simulink model "simRobotArmWith2Links"  (R2014b)
settings: Solver=ode5  StartTime=0.0  StopTime=tf  FixedStep=dt  MaxStep=dtmax  RelTol=1e-3
values from neighbouring files (symbols this model uses):
  alpha = 1    [robotArmWith2Links.m]    (also in threeLinkFTC.m; twoLinkFTC.m; twoLinkFTCwAdaptive.m)
  Ar = [0 5; -30 -30]    [robotArmWith2Links.m]    (also in threeLinkFTC.m = [0 1; -5 -5]; twoLinkFTC.m = [0 10; -40 -40]; twoLinkFTCwAdaptive.m = [0 5; -250 -250])
  Arm1 = [0 1; -wn^2 -2*ksi*wn]    [robotArmWith2Links.m]    (also in threeLinkFTC.m; twoLinkFTC.m; twoLinkFTCwAdaptive.m)
  Bfault = [0 0; 0 1]    [robotArmWith2Links.m]    (also in threeLinkFTC.m; twoLinkFTC.m; twoLinkFTCwAdaptive.m)
  Brm1 = [0 wn^2]'    [robotArmWith2Links.m]    (also in threeLinkFTC.m; twoLinkFTC.m; twoLinkFTCwAdaptive.m)
  dt = 1e-3    (= 0.001)    [robotArmWith2Links.m]
  dtFC = dt    (= 0.001)    [robotArmWith2Links.m]
  epsilon = 0.5    [robotArmWith2Links.m]    (also in threeLinkFTC.m; twoLinkFTC.m; twoLinkFTCwAdaptive.m)
  g = 9.81    [robotArmWith2Links.m]    (also in threeLinkFTC.m; twoLinkFDIbasisComparison.m; twoLinkFTC.m; twoLinkFTCwAdaptive.m)
  I1 = 8.33e-2    (= 0.0833)    [robotArmWith2Links.m]    (also in threeLinkFTC.m = 0.0833333333333; twoLinkFDIbasisComparison.m = 0.0833333333333; twoLinkFTC.m = 0.0833333333333; twoLinkFTCwAdaptive.m = 0.0833333333333)
  I2 = 8.33e-2    (= 0.0833)    [robotArmWith2Links.m]    (also in threeLinkFTC.m = 0.0833333333333; twoLinkFDIbasisComparison.m = 0.0833333333333; twoLinkFTC.m = 0.0833333333333; twoLinkFTCwAdaptive.m = 0.0833333333333)
  K1 = 2*wn*ksi    (= 87.9645943005)    [robotArmWith2Links.m]    (also in threeLinkFTC.m = 8.79645943005; twoLinkFTC.m; twoLinkFTCwAdaptive.m = 43.9822971503)
  K2 = wn^2    (= 986.960440109)    [robotArmWith2Links.m]    (also in threeLinkFTC.m = 39.4784176044; twoLinkFTC.m; twoLinkFTCwAdaptive.m)
  l1 = 1    [robotArmWith2Links.m]    (also in threeLinkFTC.m; twoLinkFDIbasisComparison.m; twoLinkFTC.m; twoLinkFTCwAdaptive.m)
  l2 = 1    [robotArmWith2Links.m]    (also in threeLinkFTC.m; twoLinkFDIbasisComparison.m; twoLinkFTC.m; twoLinkFTCwAdaptive.m)
  lc1 = l1/2    (= 0.5)    [robotArmWith2Links.m]    (also in threeLinkFTC.m; twoLinkFDIbasisComparison.m; twoLinkFTC.m; twoLinkFTCwAdaptive.m)
  lc2 = l2/2    (= 0.5)    [robotArmWith2Links.m]    (also in threeLinkFTC.m; twoLinkFDIbasisComparison.m; twoLinkFTC.m; twoLinkFTCwAdaptive.m)
  m1 = 1    [robotArmWith2Links.m]    (also in threeLinkFTC.m; twoLinkFDIbasisComparison.m; twoLinkFTC.m; twoLinkFTCwAdaptive.m)
  m2 = 1    [robotArmWith2Links.m]    (also in threeLinkFTC.m; twoLinkFDIbasisComparison.m; twoLinkFTC.m; twoLinkFTCwAdaptive.m)
  q0 = [80 20]'*pi/180    [robotArmWith2Links.m]    (also in threeLinkFTC.m = [90 0 0]'*pi/180; twoLinkFDIbasisComparison.m = [90 0]'*pi/180; twoLinkFTC.m = [90 0]'*pi/180; twoLinkFTCwAdaptive.m = [90 0]'*pi/180)
  qdot0 = [0 0]'    [robotArmWith2Links.m]    (also in threeLinkFTC.m = [0 0 0]'*pi/180; twoLinkFDIbasisComparison.m = [0 0]'*pi/180; twoLinkFTC.m = [0 0]'*pi/180; twoLinkFTCwAdaptive.m = [0 0]'*pi/180)
  r0 = [0 0]'    [robotArmWith2Links.m]    (also in threeLinkFTC.m; twoLinkFTC.m; twoLinkFTCwAdaptive.m)
  rmax = inf*[50*pi/180 inf]'    [robotArmWith2Links.m]    (also in threeLinkFTC.m; twoLinkFTC.m; twoLinkFTCwAdaptive.m)
  rmin = -rmax    [robotArmWith2Links.m]    (also in threeLinkFTC.m; twoLinkFTC.m; twoLinkFTCwAdaptive.m)
  visualFlag = 0    [robotArmWith2Links.m]    (also in twoLinkFDIbasisComparison.m; twoLinkFTC.m; twoLinkFTCwAdaptive.m)
  visualizationDataFlag = 1    [robotArmWith2Links.m]    (also in twoLinkFDIbasisComparison.m; twoLinkFTC.m; twoLinkFTCwAdaptive.m)
undefined symbols (not defined in the file or in its folder): twolinkplot
libraries: simulink x1
(part 2 of 2)

== system simRobotArmWith2Links/Controller/ FTC Controller/System model/Modelled Plant/get Plant Parameters ==
  H : Inport
  C : Inport  Port=2
  G : Inport  Port=3
  qdot : Inport  Port=4
  {1,5,7,11} (4 alike) : Selector  NumberOfDimensions=2  InputPortWidth=3  IndexOptions=Index vector (dialog),Index vector (dialog)  Indices=1,1  OutputSizes=1,1
  12 : Selector  NumberOfDimensions=2  InputPortWidth=3  IndexOptions=Index vector (dialog),Index vector (dialog)  Indices=1,2  OutputSizes=1,1
  2 : Selector  NumberOfDimensions=2  InputPortWidth=3  IndexOptions=Index vector (dialog),Index vector (dialog)  Indices=1,2  OutputSizes=1,1
  {3,6,8,21} (4 alike) : Selector  NumberOfDimensions=2  InputPortWidth=3  IndexOptions=Index vector (dialog),Index vector (dialog)  Indices=2,1  OutputSizes=1,1
  22 : Selector  NumberOfDimensions=2  InputPortWidth=3  IndexOptions=Index vector (dialog),Index vector (dialog)  Indices=2,2  OutputSizes=1,1
  4 : Selector  NumberOfDimensions=2  InputPortWidth=3  IndexOptions=Index vector (dialog),Index vector (dialog)  Indices=2,2  OutputSizes=1,1
  Bus Creator : BusCreator  Inputs=15
  Product5 : Product  Multiplication=Matrix(*)  RndMeth=Zero
  Sum of Elements1 : Sum
  busData : Outport
  wires:
  2/1 -> Bus Creator/9  "C12"
  21/1 -> Bus Creator/6  "H21"
  22/1 -> Bus Creator/7  "H22"
  4/1 -> Bus Creator/11  "C22"
  6/1 -> Bus Creator/13  "G_2"
  1/1 -> Bus Creator/8  "C11"
  5/1 -> Bus Creator/12  "G_1"
  12/1 -> Bus Creator/5  "H12"
  3/1 -> Bus Creator/10  "C21"
  11/1 -> Bus Creator/4  "H11"
  [H] -> 11/1, 12/1, 21/1, 22/1
  [C] -> 1/1, 2/1, 4/1, 3/1
  [G] -> 6/1, 5/1
  [C] -> Product5/1
  [qdot] -> Product5/2
  Product5/1 -> Sum of Elements1/1
  [G] -> Sum of Elements1/2
  Sum of Elements1/1 -> 7/1, 8/1
  7/1 -> Bus Creator/14  "phi1"
  8/1 -> Bus Creator/15  "phi2"
  [G] -> Bus Creator/3
  Bus Creator/1 -> busData/1
  [C] -> Bus Creator/2
  [H] -> Bus Creator/1
  H/1 -> [H]  "H"
  C/1 -> [C]  "C"
  G/1 -> [G]  "G"
  qdot/1 -> [qdot]

== system simRobotArmWith2Links/Controller/ FTC Controller/System model/Modelled Plant/getC ==
  s2 : Inport
  q1dot : Inport  Port=2
  q2dot : Inport  Port=3
  C calculation 1 : Subsystem
  C calculation 2 : Subsystem
  Gain2 : Gain  Gain=m2*l1*lc2
  Terminator : Terminator
  C : Outport
  wires:
  s2/1 -> [s2]
  q1dot/1 -> [q1dot]
  q2dot/1 -> [q2dot]
  [s2] -> Gain2/1
  Gain2/1 -> [h]
  [q1dot] -> C calculation 1/1(q1dot)
  [q2dot] -> C calculation 1/2(q2dot)
  [h] -> C calculation 1/3(h)
  [q1dot] -> C calculation 2/1(q1dot)
  [q2dot] -> C calculation 2/2(q2dot)
  [h] -> C calculation 2/3(h)
  [C] -> C/1
  C calculation 2/1(C) -> [C]
  C calculation 1/1(C) -> Terminator/1

== system simRobotArmWith2Links/Controller/ FTC Controller/System model/Modelled Plant/getG ==
  c1 : Inport
  c12 : Inport  Port=2
  Add : Sum
  Gain : Gain  Gain=(m1*lc1+m2*l1)*g
  Gain1 : Gain  Gain=m2*g*lc2
  Gain2 : Gain
  Gain4 : Gain  Gain=lc2*m2*g
  Matrix Concatenate2 : Concatenate  Mode=Multidimensional array
  G : Outport
  wires:
  [c12] -> Gain4/1
  Gain4/1 -> [G21]
  c12/1 -> [c12]
  c1/1 -> [c1]
  Matrix Concatenate2/1 -> Gain2/1
  [G11] -> Matrix Concatenate2/1
  [G21] -> Matrix Concatenate2/2
  [c1] -> Gain/1
  Gain/1 -> Add/1
  [c12] -> Gain1/1
  Gain1/1 -> Add/2
  Add/1 -> [G11]
  Gain2/1 -> G/1

== system simRobotArmWith2Links/Controller/ FTC Controller/System model/Modelled Plant/getH ==
  c2 : Inport
  Constant1 : Constant  Value=I1 + I2 + m1*lc1^2 + m2*(l1^2+lc2^2)  VectorParams1D=off
  Constant2 : Constant  Value=I2+m2*lc2^2  VectorParams1D=off
  Constant3 : Constant  Value=I2+m2*lc2^2  VectorParams1D=off
  Gain : Gain  Gain=m2*2*l1*lc2
  Gain1 : Gain  Gain=m2*l1*lc2
  Matrix Concatenate : Concatenate  Mode=Multidimensional array  ConcatenateDimension=2
  Matrix Concatenate1 : Concatenate  Mode=Multidimensional array  ConcatenateDimension=2
  Matrix Concatenate2 : Concatenate  Mode=Multidimensional array
  Sum : Sum
  Sum1 : Sum
  H : Outport
  wires:
  [H11] -> Matrix Concatenate/1
  [H12] -> Matrix Concatenate/2
  Matrix Concatenate/1 -> Matrix Concatenate2/1
  Matrix Concatenate1/1 -> Matrix Concatenate2/2
  [H21] -> Matrix Concatenate1/1
  [H22] -> Matrix Concatenate1/2
  Matrix Concatenate2/1 -> H/1
  c2/1 -> [c2]
  [c2] -> Gain/1
  Gain/1 -> Sum/1
  Constant1/1 -> Sum/2
  Sum/1 -> [H11]
  [c2] -> Gain1/1
  Gain1/1 -> Sum1/1
  Constant2/1 -> Sum1/2
  Sum1/1 -> [H12], [H21]
  Constant3/1 -> [H22]

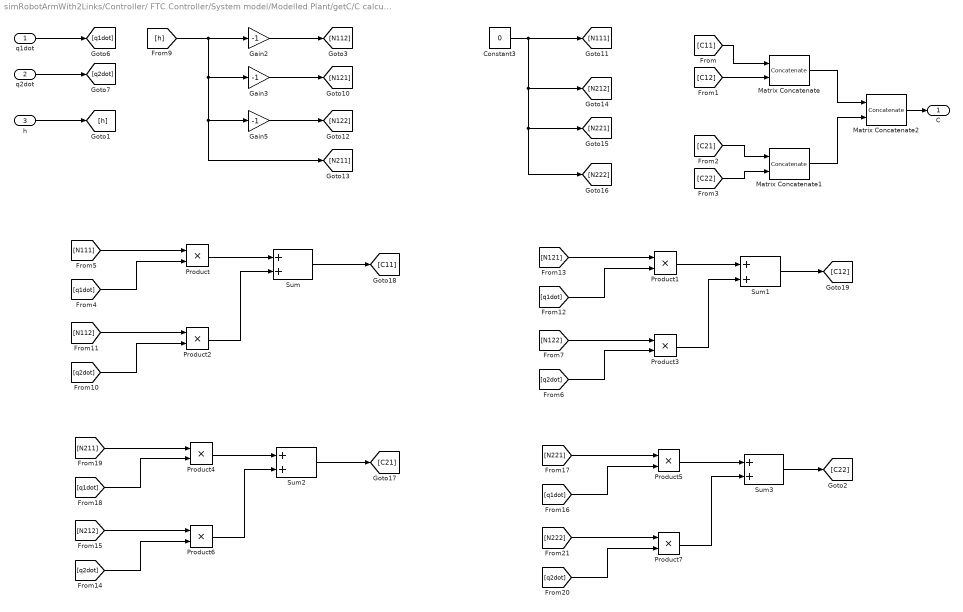
== system simRobotArmWith2Links/Controller/ FTC Controller/System model/Modelled Plant/getC/C calculation 1 ==
  q1dot : Inport
  q2dot : Inport  Port=2
  h : Inport  Port=3
  Constant3 : Constant  Value=0  VectorParams1D=off
  Gain2 : Gain  Gain=-1
  Gain3 : Gain  Gain=-1
  Gain5 : Gain  Gain=-1
  Matrix Concatenate : Concatenate  Mode=Multidimensional array  ConcatenateDimension=2
  Matrix Concatenate1 : Concatenate  Mode=Multidimensional array  ConcatenateDimension=2
  Matrix Concatenate2 : Concatenate  Mode=Multidimensional array
  Product{,1..7} (8 alike) : Product  RndMeth=Zero
  Sum{,1..3} (4 alike) : Sum
  C : Outport
  wires:
  q2dot/1 -> [q2dot]
  q1dot/1 -> [q1dot]
  [N111] -> Product/1
  Product/1 -> Sum/1
  [q1dot] -> Product/2
  [N112] -> Product2/1
  Product2/1 -> Sum/2
  [q2dot] -> Product2/2
  Sum/1 -> [C11]
  [N121] -> Product1/1
  Product1/1 -> Sum1/1
  [q1dot] -> Product1/2
  [N122] -> Product3/1
  Product3/1 -> Sum1/2
  [q2dot] -> Product3/2
  Sum1/1 -> [C12]
  [N211] -> Product4/1
  Product4/1 -> Sum2/1
  [q1dot] -> Product4/2
  [N212] -> Product6/1
  Product6/1 -> Sum2/2
  [q2dot] -> Product6/2
  Sum2/1 -> [C21]
  [N221] -> Product5/1
  Product5/1 -> Sum3/1
  [q1dot] -> Product5/2
  [N222] -> Product7/1
  Product7/1 -> Sum3/2
  [q2dot] -> Product7/2
  Constant3/1 -> [N111], [N212], [N221], [N222]
  [h] -> Gain2/1, Gain3/1, Gain5/1, [N211]
  Gain2/1 -> [N112]
  Gain3/1 -> [N121]
  Gain5/1 -> [N122]
  h/1 -> [h]
  Sum3/1 -> [C22]
  Matrix Concatenate2/1 -> C/1
  [C22] -> Matrix Concatenate1/2
  [C21] -> Matrix Concatenate1/1
  Matrix Concatenate1/1 -> Matrix Concatenate2/2
  Matrix Concatenate/1 -> Matrix Concatenate2/1
  [C12] -> Matrix Concatenate/2
  [C11] -> Matrix Concatenate/1

== system simRobotArmWith2Links/Controller/ FTC Controller/System model/Modelled Plant/getC/C calculation 2 ==
  q1dot : Inport
  q2dot : Inport  Port=2
  h : Inport  Port=3
  Constant1 : Constant  Value=0  VectorParams1D=off
  Gain6 : Gain  Gain=-2
  Gain7 : Gain  Gain=-1
  Matrix Concatenate : Concatenate  Mode=Multidimensional array  ConcatenateDimension=2
  Matrix Concatenate1 : Concatenate  Mode=Multidimensional array  ConcatenateDimension=2
  Matrix Concatenate2 : Concatenate  Mode=Multidimensional array
  Product10 : Product  RndMeth=Zero
  Product8 : Product  RndMeth=Zero
  Product9 : Product  RndMeth=Zero
  C : Outport
  wires:
  h/1 -> [h]
  q1dot/1 -> [q1dot]
  q2dot/1 -> [q2dot]
  [h] -> Gain6/1
  [h] -> Gain7/1
  Gain7/1 -> Product10/2
  Product10/1 -> [C12]
  Constant1/1 -> [C22]
  [h] -> Product8/2
  [q1dot] -> Product8/1
  Product8/1 -> [C21]
  Gain6/1 -> Product9/2
  Product9/1 -> [C11]
  [q2dot] -> Product9/1
  Matrix Concatenate2/1 -> C/1
  [C22] -> Matrix Concatenate1/2
  [C21] -> Matrix Concatenate1/1
  Matrix Concatenate1/1 -> Matrix Concatenate2/2
  Matrix Concatenate/1 -> Matrix Concatenate2/1
  [C12] -> Matrix Concatenate/2
  [C11] -> Matrix Concatenate/1
  [q2dot] -> Product10/1
